simulink model "Application_Problem_Solution"  (R2018b)
settings: Solver=VariableStepAuto  StartTime=0.0  StopTime=6300  FixedStep=0.1  RelTol=1e-3  EnableMultiTasking=on
StopFcn:
  | if sum(Diagnostic_Decision_PV_1)>0
  | f = msgbox('Failure in PV 1');
  | end
  | 
  | if sum(Diagnostic_Decision_PV_2)>0
  | f = msgbox('Failure in PV 2');
  | end
  | 
  | if sum(Diagnostic_Decision_PV_3)>0
  | f = msgbox('Failure in PV 3');
  | end
  | 
  | if sum(Diagnostic_Decision_PV_4)>0
  | f = msgbox('Failure in PV 4');
  | end
  | 
  | if sum(Diagnostic_Decision_PV_5)>0
  | f = msgbox('Failure in PV 5');
  | end
  | 
  | if sum(Diagnostic_Decision_PV_6)>0
  | f = msgbox('Failure in PV 6');
  | end
  | 
  | if sum(Diagnostic_Decision_PV_7)>0
  | f = msgbox('Failure in PV 7');
  | end
  | 
  | if sum(Diagnostic_Decision_PV_8)>0
  | f = msgbox('Failure in PV 8');
  | end
  | 
  | if sum(Diagnostic_Decision_PV_9)>0
  | f = msgbox('Failure in PV 9');
  | end
  | 
  | if sum(Diagnostic_Decision_PV_10)>0
  | f = msgbox('Failure in PV 10');
  | end
values from neighbouring files (symbols this model uses):
  C1_LUT = [1913.6 4625.7 23306 10736 18036 12251 9022.9 12447 18872 40764 18721 33630 ... (21 elements, 7x3)]    [model_data_application.mat]
  Capacity_LUT = [28.0081 27.625 27.6392]    [model_data_application.mat]
  cell_Cp_heat = 810.5328    [model_data_application.mat]
  cell_mass = 1    [model_data_application.mat]
  Em_LUT = [3.4966 3.5519 3.6183 3.7066 3.9131 4.0748 4.1923 3.5057 3.566 3.6337 3.7127 3.9259 ... (21 elements, 7x3)]    [model_data_application.mat]
  Qe_init = 3.6845    [model_data_application.mat]
  R0_LUT = [0.0117 0.011 0.0114 0.0107 0.0107 0.0113 0.0116 0.0085 0.0085 0.0087 0.0082 0.0083 ... (21 elements, 7x3)]    [model_data_application.mat]
  R1_LUT = [0.0109 0.0069 0.0047 0.0034 0.0033 0.0033 0.0028 0.0029 0.0024 0.0026 0.0016 0.0023 ... (21 elements, 7x3)]    [model_data_application.mat]
  SOC_LUT = [0 0.1 0.25 0.5 0.75 0.9 1]    [model_data_application.mat]
  T_init = 293.15    [model_data_application.mat]
  Temperature_LUT = [278.15 293.15 313.15]    [model_data_application.mat]
undefined symbols (not defined in the file or in its folder): DiscIntNeverNeededParam
libraries: elec_lib x450, fl_lib x121, LiBatteryElements_lib x40, nesl_utility x32, simulink x10
(part 2 of 3)

== system Application_Problem_Solution/Battery7 ==
  C1 : LiBatteryElements_lib/C_table  C_Table=C1_LUT F  SOC_Table=SOC_LUT  Temp_Table=Temperature_LUT K  v0=0 V
  Convective Heat Transfer : fl_lib/Thermal/Thermal Elements/Convective Heat Transfer  area=cell_area m^2  heat_tr_coeff=h_conv W/(m^2 * K)  T_specify=off  T_priority=High  T=0 K  T_nominal_specify=off  T_nominal_unit=K  T_nominal_value=1  Q_specify=off  Q_priority=High  Q=0 J/s  Q_nominal_specify=off  Q_nominal_unit=W  Q_nominal_value=1
  Em_table : LiBatteryElements_lib/Em_table  C_Table=Capacity_LUT hr*A  Em_Table=Em_LUT V  SOC_Table=SOC_LUT  Temp_Table=Temperature_LUT K  Qinit=Qe_init hr*A
  Ideal Temperature Source : fl_lib/Thermal/Thermal Sources/Controlled Temperature Source
      settings: SourceProductName=Simscape
  Power Sum : fl_lib/Physical Signals/Functions/PS Add
  R0 : LiBatteryElements_lib/R_table  R_Table=R0_LUT Ohm  SOC_Table=SOC_LUT  Temp_Table=Temperature_LUT K
  R1 : LiBatteryElements_lib/R_table  R_Table=R1_LUT Ohm  SOC_Table=SOC_LUT  Temp_Table=Temperature_LUT K
  Simulink-PS Converter2 : nesl_utility/Simulink-PS Converter  PhysicalDomain=network_engine_domain  SubClassName=ps_input  LeftPortType=input  RightPortType=output  PseudoPeriodic=off  Frequencies=[]  NoiseDistribution=none  NoiseParameters=[]  Unit=degC  AffineConversion=on  FilteringAndDerivatives=zero  SimscapeFilterOrder=1  InputFilterTimeConstant=.001  UdotUserProvided=1
  Thermal Model : Subsystem
  Thermal Reference : fl_lib/Thermal/Thermal Elements/Thermal Reference
  temp : Constant  Value=25
  + : PMIOPort  Tag=PMCPort  Side=Left
  - : PMIOPort  Tag=PMCPort  Port=2  Side=Right
  wires:
  temp/1 -> Simulink-PS Converter2/1
  connections:
  Thermal Reference/LConn1 -- Ideal Temperature Source/RConn2
  Ideal Temperature Source/LConn1 -- Convective Heat Transfer/LConn1
  Simulink-PS Converter2/RConn1 -- Ideal Temperature Source/RConn1
  R0/RConn2 -- Power Sum/LConn1
  R0/LConn1 -- C1/RConn1 -- R1/RConn1
  Power Sum/RConn1 -- Thermal Model/LConn1
  C1/LConn2 -- R0/LConn2 -- Em_table/RConn2 -- Thermal Model/RConn1 -- R1/LConn2
  R1/RConn2 -- Power Sum/LConn2
  R1/LConn1 -- C1/LConn1 -- Em_table/LConn1
  +/RConn1 -- R0/RConn1
  Em_table/RConn1 -- -/RConn1
  Convective Heat Transfer/RConn1 -- Thermal Model/LConn2
  C1/LConn3 -- Em_table/LConn3 -- R0/LConn3 -- R1/LConn3

== system Application_Problem_Solution/Battery8 ==
  C1 : LiBatteryElements_lib/C_table  C_Table=C1_LUT F  SOC_Table=SOC_LUT  Temp_Table=Temperature_LUT K  v0=0 V
  Convective Heat Transfer : fl_lib/Thermal/Thermal Elements/Convective Heat Transfer  area=cell_area m^2  heat_tr_coeff=h_conv W/(m^2 * K)  T_specify=off  T_priority=High  T=0 K  T_nominal_specify=off  T_nominal_unit=K  T_nominal_value=1  Q_specify=off  Q_priority=High  Q=0 J/s  Q_nominal_specify=off  Q_nominal_unit=W  Q_nominal_value=1
  Em_table : LiBatteryElements_lib/Em_table  C_Table=Capacity_LUT hr*A  Em_Table=Em_LUT V  SOC_Table=SOC_LUT  Temp_Table=Temperature_LUT K  Qinit=Qe_init hr*A
  Ideal Temperature Source : fl_lib/Thermal/Thermal Sources/Controlled Temperature Source
      settings: SourceProductName=Simscape
  Power Sum : fl_lib/Physical Signals/Functions/PS Add
  R0 : LiBatteryElements_lib/R_table  R_Table=R0_LUT Ohm  SOC_Table=SOC_LUT  Temp_Table=Temperature_LUT K
  R1 : LiBatteryElements_lib/R_table  R_Table=R1_LUT Ohm  SOC_Table=SOC_LUT  Temp_Table=Temperature_LUT K
  Simulink-PS Converter2 : nesl_utility/Simulink-PS Converter  PhysicalDomain=network_engine_domain  SubClassName=ps_input  LeftPortType=input  RightPortType=output  PseudoPeriodic=off  Frequencies=[]  NoiseDistribution=none  NoiseParameters=[]  Unit=degC  AffineConversion=on  FilteringAndDerivatives=zero  SimscapeFilterOrder=1  InputFilterTimeConstant=.001  UdotUserProvided=1
  Thermal Model : Subsystem
  Thermal Reference : fl_lib/Thermal/Thermal Elements/Thermal Reference
  temp : Constant  Value=25
  + : PMIOPort  Tag=PMCPort  Side=Left
  - : PMIOPort  Tag=PMCPort  Port=2  Side=Right
  wires:
  temp/1 -> Simulink-PS Converter2/1
  connections:
  R1/LConn3 -- R0/LConn3 -- Em_table/LConn3 -- C1/LConn3
  Convective Heat Transfer/RConn1 -- Thermal Model/LConn2
  Em_table/RConn1 -- -/RConn1
  +/RConn1 -- R0/RConn1
  Em_table/LConn1 -- C1/LConn1 -- R1/LConn1
  R1/RConn2 -- Power Sum/LConn2
  R1/LConn2 -- Thermal Model/RConn1 -- Em_table/RConn2 -- R0/LConn2 -- C1/LConn2
  Power Sum/RConn1 -- Thermal Model/LConn1
  R1/RConn1 -- C1/RConn1 -- R0/LConn1
  R0/RConn2 -- Power Sum/LConn1
  Simulink-PS Converter2/RConn1 -- Ideal Temperature Source/RConn1
  Ideal Temperature Source/LConn1 -- Convective Heat Transfer/LConn1
  Thermal Reference/LConn1 -- Ideal Temperature Source/RConn2

== system Application_Problem_Solution/Battery9 ==
  C1 : LiBatteryElements_lib/C_table  C_Table=C1_LUT F  SOC_Table=SOC_LUT  Temp_Table=Temperature_LUT K  v0=0 V
  Convective Heat Transfer : fl_lib/Thermal/Thermal Elements/Convective Heat Transfer  area=cell_area m^2  heat_tr_coeff=h_conv W/(m^2 * K)  T_specify=off  T_priority=High  T=0 K  T_nominal_specify=off  T_nominal_unit=K  T_nominal_value=1  Q_specify=off  Q_priority=High  Q=0 J/s  Q_nominal_specify=off  Q_nominal_unit=W  Q_nominal_value=1
  Em_table : LiBatteryElements_lib/Em_table  C_Table=Capacity_LUT hr*A  Em_Table=Em_LUT V  SOC_Table=SOC_LUT  Temp_Table=Temperature_LUT K  Qinit=Qe_init hr*A
  Ideal Temperature Source : fl_lib/Thermal/Thermal Sources/Controlled Temperature Source
      settings: SourceProductName=Simscape
  Power Sum : fl_lib/Physical Signals/Functions/PS Add
  R0 : LiBatteryElements_lib/R_table  R_Table=R0_LUT Ohm  SOC_Table=SOC_LUT  Temp_Table=Temperature_LUT K
  R1 : LiBatteryElements_lib/R_table  R_Table=R1_LUT Ohm  SOC_Table=SOC_LUT  Temp_Table=Temperature_LUT K
  Simulink-PS Converter2 : nesl_utility/Simulink-PS Converter  PhysicalDomain=network_engine_domain  SubClassName=ps_input  LeftPortType=input  RightPortType=output  PseudoPeriodic=off  Frequencies=[]  NoiseDistribution=none  NoiseParameters=[]  Unit=degC  AffineConversion=on  FilteringAndDerivatives=zero  SimscapeFilterOrder=1  InputFilterTimeConstant=.001  UdotUserProvided=1
  Thermal Model : Subsystem
  Thermal Reference : fl_lib/Thermal/Thermal Elements/Thermal Reference
  temp : Constant  Value=25
  + : PMIOPort  Tag=PMCPort  Side=Left
  - : PMIOPort  Tag=PMCPort  Port=2  Side=Right
  wires:
  temp/1 -> Simulink-PS Converter2/1
  connections:
  Thermal Reference/LConn1 -- Ideal Temperature Source/RConn2
  Ideal Temperature Source/LConn1 -- Convective Heat Transfer/LConn1
  Simulink-PS Converter2/RConn1 -- Ideal Temperature Source/RConn1
  R0/RConn2 -- Power Sum/LConn1
  R0/LConn1 -- C1/RConn1 -- R1/RConn1
  Power Sum/RConn1 -- Thermal Model/LConn1
  C1/LConn2 -- R0/LConn2 -- Em_table/RConn2 -- Thermal Model/RConn1 -- R1/LConn2
  R1/RConn2 -- Power Sum/LConn2
  R1/LConn1 -- C1/LConn1 -- Em_table/LConn1
  +/RConn1 -- R0/RConn1
  Em_table/RConn1 -- -/RConn1
  Convective Heat Transfer/RConn1 -- Thermal Model/LConn2
  C1/LConn3 -- Em_table/LConn3 -- R0/LConn3 -- R1/LConn3

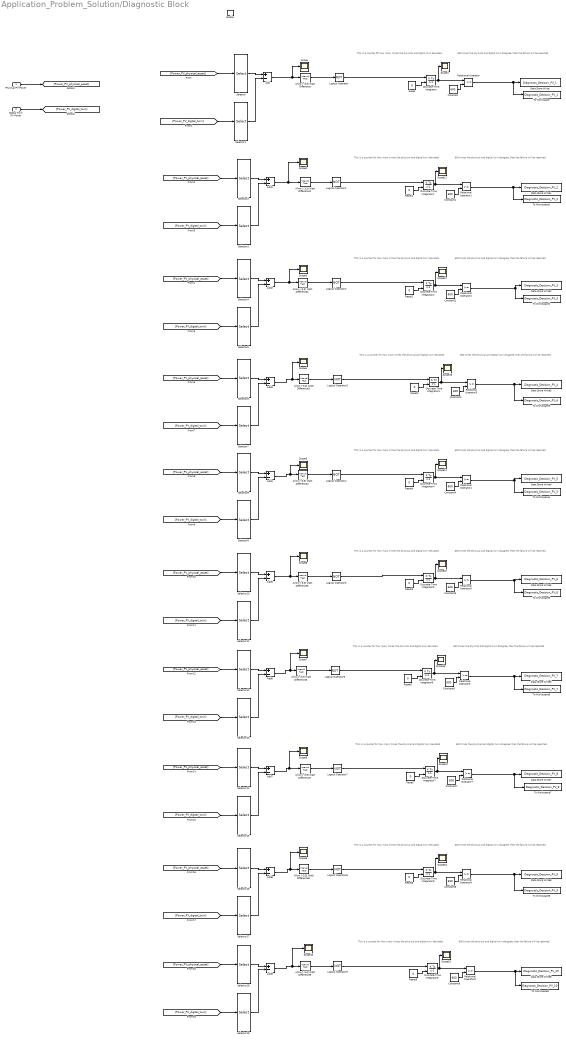
== system Application_Problem_Solution/Diagnostic Block ==
  note: 600 times the physical and digital twin disagree, then the failure will be reported.
  note: This is a counter for how many times the physical and digital twin deviated.
  note: 600 times the physical and digital twin disagree, then the failure will be reported.
  note: This is a counter for how many times the physical and digital twin deviated.
  note: 600 times the physical and digital twin disagree, then the failure will be reported.
  note: This is a counter for how many times the physical and digital twin deviated.
  note: 600 times the physical and digital twin disagree, then the failure will be reported.
  note: This is a counter for how many times the physical and digital twin deviated.
  note: 600 times the physical and digital twin disagree, then the failure will be reported.
  note: This is a counter for how many times the physical and digital twin deviated.
  note: 600 times the physical and digital twin disagree, then the failure will be reported.
  note: This is a counter for how many times the physical and digital twin deviated.
  note: 600 times the physical and digital twin disagree, then the failure will be reported.
  note: This is a counter for how many times the physical and digital twin deviated.
  note: 600 times the physical and digital twin disagree, then the failure will be reported.
  note: This is a counter for how many times the physical and digital twin deviated.
  note: 600 times the physical and digital twin disagree, then the failure will be reported.
  note: This is a counter for how many times the physical and digital twin deviated.
  note: 600 times the physical and digital twin disagree, then the failure will be reported.
  note: This is a counter for how many times the physical and digital twin deviated.
  Physical PV-Power : Inport
  Digital Twin PV-Power : Inport  Port=2
  Enable : EnablePort
  Add{,1..9} (10 alike) : Sum  Inputs=+-
  Allow [-3,3] Watt Difference{,1..9} (10 alike) : simulink/Logic and Bit Operations/Interval Test  IntervalClosedRight=on  uplimit=3  IntervalClosedLeft=on  lowlimit=-3  OutDataTypeStr=boolean
  Constant{,1..9} (10 alike) : Constant  Value=600
  Data Store Write : DataStoreWrite  DataStoreName=Diagnostic_Decision_PV_1  SampleTime=10
  Data Store Write1 : DataStoreWrite  DataStoreName=Diagnostic_Decision_PV_2  SampleTime=100
  Data Store Write2 : DataStoreWrite  DataStoreName=Diagnostic_Decision_PV_3  SampleTime=10
  Data Store Write3 : DataStoreWrite  DataStoreName=Diagnostic_Decision_PV_4  SampleTime=10
  Data Store Write4 : DataStoreWrite  DataStoreName=Diagnostic_Decision_PV_5  SampleTime=10
  Data Store Write5 : DataStoreWrite  DataStoreName=Diagnostic_Decision_PV_6
  Data Store Write6 : DataStoreWrite  DataStoreName=Diagnostic_Decision_PV_7  SampleTime=10
  Data Store Write7 : DataStoreWrite  DataStoreName=Diagnostic_Decision_PV_8  SampleTime=10
  Data Store Write8 : DataStoreWrite  DataStoreName=Diagnostic_Decision_PV_9  SampleTime=10
  Data Store Write9 : DataStoreWrite  DataStoreName=Diagnostic_Decision_PV_10  SampleTime=10
  Discrete-Time Integrator : DiscreteIntegrator  ExternalReset=rising  SampleTime=10  ICPrevOutput=DiscIntNeverNeededParam  ICPrevScaledInput=DiscIntNeverNeededParam
  Discrete-Time Integrator{1..9} (9 alike) : DiscreteIntegrator  ExternalReset=level  SampleTime=10  ICPrevOutput=DiscIntNeverNeededParam  ICPrevScaledInput=DiscIntNeverNeededParam
  Logical Operator{,1..9} (10 alike) : Logic  Operator=NOT  AllPortsSameDT=off  OutDataTypeStr=boolean
  Relational Operator{,1..9} (10 alike) : RelationalOperator  OutDataTypeStr=boolean  RndMeth=Simplest
  Reset{,1..9} (10 alike) : Constant  Value=0
  Scope{,1..19} (20 alike) : Scope
  Selector : Selector  InputPortWidth=10  IndexOptions=Index vector (dialog)  Indices=1  OutputSizes=1
  Selector1 : Selector  InputPortWidth=10  IndexOptions=Index vector (dialog)  Indices=1  OutputSizes=1
  Selector{10..13} (4 alike) : Selector  InputPortWidth=10  IndexOptions=Index vector (dialog)  Indices=6  OutputSizes=1
  Selector14 : Selector  InputPortWidth=10  IndexOptions=Index vector (dialog)  Indices=8  OutputSizes=1
  Selector15 : Selector  InputPortWidth=10  IndexOptions=Index vector (dialog)  Indices=8  OutputSizes=1
  Selector16 : Selector  InputPortWidth=10  IndexOptions=Index vector (dialog)  Indices=9  OutputSizes=1
  Selector17 : Selector  InputPortWidth=10  IndexOptions=Index vector (dialog)  Indices=9  OutputSizes=1
  Selector18 : Selector  InputPortWidth=10  IndexOptions=Index vector (dialog)  Indices=10  OutputSizes=1
  Selector19 : Selector  InputPortWidth=10  IndexOptions=Index vector (dialog)  Indices=10  OutputSizes=1
  Selector2 : Selector  InputPortWidth=10  IndexOptions=Index vector (dialog)  Indices=2  OutputSizes=1
  Selector3 : Selector  InputPortWidth=10  IndexOptions=Index vector (dialog)  Indices=2  OutputSizes=1
  Selector4 : Selector  InputPortWidth=10  IndexOptions=Index vector (dialog)  Indices=3  OutputSizes=1
  Selector5 : Selector  InputPortWidth=10  IndexOptions=Index vector (dialog)  Indices=3  OutputSizes=1
  Selector6 : Selector  InputPortWidth=10  IndexOptions=Index vector (dialog)  Indices=4  OutputSizes=1
  Selector7 : Selector  InputPortWidth=10  IndexOptions=Index vector (dialog)  Indices=4  OutputSizes=1
  Selector8 : Selector  InputPortWidth=10  IndexOptions=Index vector (dialog)  Indices=5  OutputSizes=1
  Selector9 : Selector  InputPortWidth=10  IndexOptions=Index vector (dialog)  Indices=5  OutputSizes=1
  To Workspace : ToWorkspace  VariableName=Diagnostic_Decision_PV_1  SampleTime=10
  To Workspace1 : ToWorkspace  VariableName=Diagnostic_Decision_PV_2  SampleTime=10
  To Workspace2 : ToWorkspace  VariableName=Diagnostic_Decision_PV_3  SampleTime=10
  To Workspace3 : ToWorkspace  VariableName=Diagnostic_Decision_PV_4  SampleTime=10
  To Workspace4 : ToWorkspace  VariableName=Diagnostic_Decision_PV_5  SampleTime=10
  To Workspace5 : ToWorkspace  VariableName=Diagnostic_Decision_PV_6  SampleTime=10
  To Workspace6 : ToWorkspace  VariableName=Diagnostic_Decision_PV_7  SampleTime=10
  To Workspace7 : ToWorkspace  VariableName=Diagnostic_Decision_PV_8  SampleTime=10
  To Workspace8 : ToWorkspace  VariableName=Diagnostic_Decision_PV_9  SampleTime=10
  To Workspace9 : ToWorkspace  VariableName=Diagnostic_Decision_PV_10  SampleTime=10
  wires:
  Physical PV-Power/1 -> [Power_PV_physical_asset]
  Digital Twin PV-Power/1 -> [Power_PV_digital_twin]
  [Power_PV_physical_asset] -> Selector/1
  [Power_PV_digital_twin] -> Selector1/1
  Selector/1 -> Add/1
  Selector1/1 -> Add/2
  Discrete-Time Integrator/1 -> Scope1/1, Relational Operator/1
  Constant/1 -> Relational Operator/2
  Relational Operator/1 -> To Workspace/1, Data Store Write/1
  Selector3/1 -> Add1/2
  Selector2/1 -> Add1/1
  [Power_PV_digital_twin] -> Selector3/1
  [Power_PV_physical_asset] -> Selector2/1
  [Power_PV_physical_asset] -> Selector4/1
  [Power_PV_digital_twin] -> Selector5/1
  Selector4/1 -> Add2/1
  Selector5/1 -> Add2/2
  Selector7/1 -> Add3/2
  Selector6/1 -> Add3/1
  [Power_PV_digital_twin] -> Selector7/1
  [Power_PV_physical_asset] -> Selector6/1
  [Power_PV_physical_asset] -> Selector8/1
  [Power_PV_digital_twin] -> Selector9/1
  Selector8/1 -> Add4/1
  Selector9/1 -> Add4/2
  Selector11/1 -> Add5/2
  Selector10/1 -> Add5/1
  [Power_PV_digital_twin] -> Selector11/1
  [Power_PV_physical_asset] -> Selector10/1
  [Power_PV_physical_asset] -> Selector12/1
  [Power_PV_digital_twin] -> Selector13/1
  Selector12/1 -> Add6/1
  Selector13/1 -> Add6/2
  Selector15/1 -> Add7/2
  Selector14/1 -> Add7/1
  [Power_PV_digital_twin] -> Selector15/1
  [Power_PV_physical_asset] -> Selector14/1
  [Power_PV_physical_asset] -> Selector16/1
  [Power_PV_digital_twin] -> Selector17/1
  Selector16/1 -> Add8/1
  Selector17/1 -> Add8/2
  Selector19/1 -> Add9/2
  Selector18/1 -> Add9/1
  [Power_PV_digital_twin] -> Selector19/1
  [Power_PV_physical_asset] -> Selector18/1
  Add/1 -> Scope/1, Allow [-3,3] Watt Difference/1
  Allow [-3,3] Watt Difference/1 -> Logical Operator/1
  Logical Operator/1 -> Discrete-Time Integrator/1
  Allow [-3,3] Watt Difference1/1 -> Logical Operator1/1
  Add1/1 -> Allow [-3,3] Watt Difference1/1, Scope2/1
  Add2/1 -> Allow [-3,3] Watt Difference2/1, Scope3/1
  Allow [-3,3] Watt Difference2/1 -> Logical Operator2/1
  Add3/1 -> Allow [-3,3] Watt Difference3/1, Scope4/1
  Allow [-3,3] Watt Difference3/1 -> Logical Operator3/1
  Add4/1 -> Scope5/1, Allow [-3,3] Watt Difference4/1
  Allow [-3,3] Watt Difference4/1 -> Logical Operator4/1
  Add5/1 -> Allow [-3,3] Watt Difference5/1, Scope6/1
  Allow [-3,3] Watt Difference5/1 -> Logical Operator5/1
  Add6/1 -> Scope7/1, Allow [-3,3] Watt Difference6/1
  Allow [-3,3] Watt Difference6/1 -> Logical Operator6/1
  Add7/1 -> Allow [-3,3] Watt Difference7/1, Scope8/1
  Allow [-3,3] Watt Difference7/1 -> Logical Operator7/1
  Add8/1 -> Allow [-3,3] Watt Difference8/1, Scope9/1
  Allow [-3,3] Watt Difference8/1 -> Logical Operator8/1
  Add9/1 -> Allow [-3,3] Watt Difference9/1, Scope10/1
  Allow [-3,3] Watt Difference9/1 -> Logical Operator9/1
  Reset/1 -> Discrete-Time Integrator/2
  Discrete-Time Integrator1/1 -> Scope11/1, Relational Operator1/1
  Logical Operator1/1 -> Discrete-Time Integrator1/1
  Constant1/1 -> Relational Operator1/2
  Reset1/1 -> Discrete-Time Integrator1/2
  Relational Operator1/1 -> To Workspace1/1, Data Store Write1/1
  Discrete-Time Integrator2/1 -> Scope12/1, Relational Operator2/1
  Logical Operator2/1 -> Discrete-Time Integrator2/1
  Constant2/1 -> Relational Operator2/2
  Reset2/1 -> Discrete-Time Integrator2/2
  Relational Operator2/1 -> Data Store Write2/1, To Workspace2/1
  Discrete-Time Integrator3/1 -> Scope13/1, Relational Operator3/1
  Logical Operator3/1 -> Discrete-Time Integrator3/1
  Constant3/1 -> Relational Operator3/2
  Reset3/1 -> Discrete-Time Integrator3/2
  Relational Operator3/1 -> Data Store Write3/1, To Workspace3/1
  Discrete-Time Integrator4/1 -> Scope14/1, Relational Operator4/1
  Logical Operator4/1 -> Discrete-Time Integrator4/1
  Constant4/1 -> Relational Operator4/2
  Reset4/1 -> Discrete-Time Integrator4/2
  Relational Operator4/1 -> Data Store Write4/1, To Workspace4/1
  Discrete-Time Integrator5/1 -> Scope15/1, Relational Operator5/1
  Logical Operator5/1 -> Discrete-Time Integrator5/1
  Constant5/1 -> Relational Operator5/2
  Reset5/1 -> Discrete-Time Integrator5/2
  Relational Operator5/1 -> Data Store Write5/1, To Workspace5/1
  Discrete-Time Integrator6/1 -> Scope16/1, Relational Operator6/1
  Logical Operator6/1 -> Discrete-Time Integrator6/1
  Constant6/1 -> Relational Operator6/2
  Reset6/1 -> Discrete-Time Integrator6/2
  Relational Operator6/1 -> To Workspace6/1, Data Store Write6/1
  Discrete-Time Integrator7/1 -> Scope17/1, Relational Operator7/1
  Logical Operator7/1 -> Discrete-Time Integrator7/1
  Constant7/1 -> Relational Operator7/2
  Reset7/1 -> Discrete-Time Integrator7/2
  Relational Operator7/1 -> To Workspace7/1, Data Store Write7/1
  Discrete-Time Integrator8/1 -> Scope18/1, Relational Operator8/1
  Logical Operator8/1 -> Discrete-Time Integrator8/1
  Constant8/1 -> Relational Operator8/2
  Reset8/1 -> Discrete-Time Integrator8/2
  Relational Operator8/1 -> To Workspace8/1, Data Store Write8/1
  Discrete-Time Integrator9/1 -> Scope19/1, Relational Operator9/1
  Logical Operator9/1 -> Discrete-Time Integrator9/1
  Constant9/1 -> Relational Operator9/2
  Reset9/1 -> Discrete-Time Integrator9/2
  Relational Operator9/1 -> Data Store Write9/1, To Workspace9/1

== system Application_Problem_Solution/PV 1 Physical ==
  note: 'This is a dummy model for the physical system. It is used for display reasons. Data has been pre-generated.'
  In1 : Inport
  Power_PV1_physical_asset : FromWorkspace  VariableName=Power_PV1_physical_asset  SampleTime=0
  Terminator : Terminator
  Out1 : Outport
  wires:
  In1/1 -> Terminator/1
  Power_PV1_physical_asset/1 -> Out1/1

== system Application_Problem_Solution/PV 10 Physical ==
  note: 'This is a dummy model for the physical system. It is used for display reasons. Data has been pre-generated.'
  In1 : Inport
  Power_PV1_physical_asset : FromWorkspace  VariableName=Power_PV10_physical_asset  SampleTime=0
  Terminator : Terminator
  Out1 : Outport
  wires:
  Power_PV1_physical_asset/1 -> Out1/1
  In1/1 -> Terminator/1

== system Application_Problem_Solution/PV 2 Physical  ==
  note: 'This is a dummy model for the physical system. It is used for display reasons. Data has been pre-generated.'
  In1 : Inport
  Power_PV2_physical_asset : FromWorkspace  VariableName=Power_PV2_physical_asset  SampleTime=0
  Terminator : Terminator
  Out1 : Outport
  wires:
  Power_PV2_physical_asset/1 -> Out1/1
  In1/1 -> Terminator/1

== system Application_Problem_Solution/PV 3 Physical ==
  note: 'This is a dummy model for the physical system. It is used for display reasons. Data has been pre-generated.'
  In1 : Inport
  Power_PV3_physical_asset : FromWorkspace  VariableName=Power_PV3_physical_asset  SampleTime=0
  Terminator : Terminator
  Out1 : Outport
  wires:
  In1/1 -> Terminator/1
  Power_PV3_physical_asset/1 -> Out1/1

== system Application_Problem_Solution/PV 4 Physical ==
  note: 'This is a dummy model for the physical system. It is used for display reasons. Data has been pre-generated.'
  In1 : Inport
  Power_PV4_physical_asset : FromWorkspace  VariableName=Power_PV4_physical_asset  SampleTime=0
  Terminator : Terminator
  Out1 : Outport
  wires:
  Power_PV4_physical_asset/1 -> Out1/1
  In1/1 -> Terminator/1

== system Application_Problem_Solution/PV 5 Physical ==
  note: 'This is a dummy model for the physical system. It is used for display reasons. Data has been pre-generated.'
  In1 : Inport
  Power_PV5_physical_asset : FromWorkspace  VariableName=Power_PV5_physical_asset  SampleTime=0
  Terminator : Terminator
  Out1 : Outport
  wires:
  In1/1 -> Terminator/1
  Power_PV5_physical_asset/1 -> Out1/1

== system Application_Problem_Solution/PV 6 Physical ==
  note: 'This is a dummy model for the physical system. It is used for display reasons. Data has been pre-generated.'
  In1 : Inport
  Power_PV6_physical_asset : FromWorkspace  VariableName=Power_PV6_physical_asset  SampleTime=0
  Terminator : Terminator
  Out1 : Outport
  wires:
  Power_PV6_physical_asset/1 -> Out1/1
  In1/1 -> Terminator/1

== system Application_Problem_Solution/PV 7 Physical ==
  note: 'This is a dummy model for the physical system. It is used for display reasons. Data has been pre-generated.'
  In1 : Inport
  Power_PV7_physical_asset : FromWorkspace  VariableName=Power_PV7_physical_asset  SampleTime=0
  Terminator : Terminator
  Out1 : Outport
  wires:
  In1/1 -> Terminator/1
  Power_PV7_physical_asset/1 -> Out1/1

== system Application_Problem_Solution/PV 8 Physical ==
  note: 'This is a dummy model for the physical system. It is used for display reasons. Data has been pre-generated.'
  In1 : Inport
  Power_PV1_physical_asset : FromWorkspace  VariableName=Power_PV8_physical_asset  SampleTime=0
  Terminator : Terminator
  Out1 : Outport
  wires:
  Power_PV1_physical_asset/1 -> Out1/1
  In1/1 -> Terminator/1

== system Application_Problem_Solution/PV 9 Physical ==
  note: 'This is a dummy model for the physical system. It is used for display reasons. Data has been pre-generated.'
  In1 : Inport
  Power_PV1_physical_asset : FromWorkspace  VariableName=Power_PV9_physical_asset  SampleTime=0
  Terminator : Terminator
  Out1 : Outport
  wires:
  In1/1 -> Terminator/1
  Power_PV1_physical_asset/1 -> Out1/1

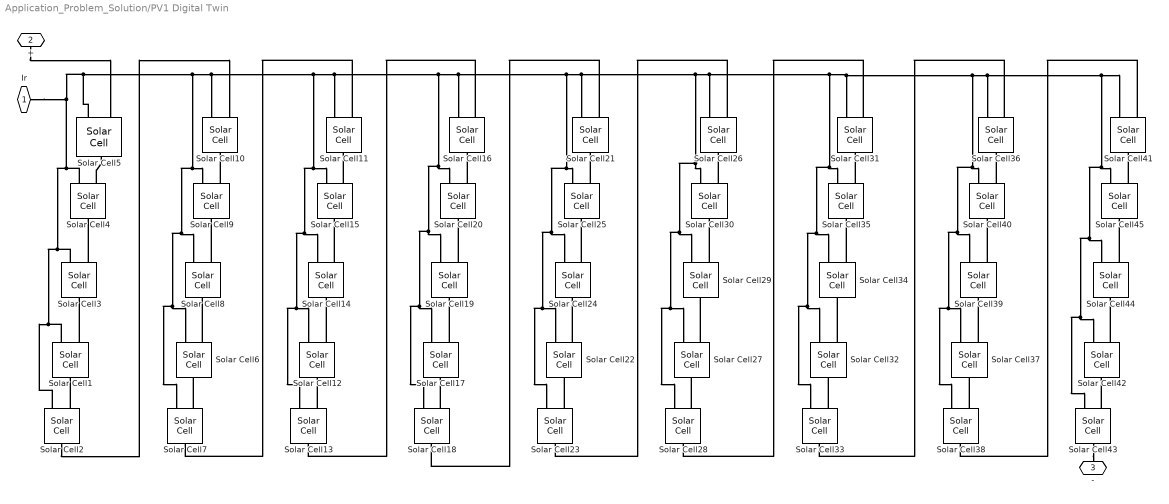
== system Application_Problem_Solution/PV1 Digital Twin ==
  Solar Cell{1..45} (45 alike) : elec_lib/Sources/Solar Cell  prm=1  Isc=Isc A  Voc=Voc/45 V  Is=1e-6 A  Is2=0 A  Iph=7.34 A  Ir0=Ir0 W/m^2  ec=n  N2=2  Rs=Rs/45 Ohm  Rp=Inf Ohm  N_series=1  TIPH1=0 1/K  EG=1.11 eV  TXIS1=3  TXIS2=3  TRS1=0  TRP1=0  Tmeas=T degC  TFIXED=T degC  thermal_mass=100 J/K  initial_temperature=25 degC
      settings: SourceProductName=Simscape Electronics  SourceProductBaseCode=SN
  Ir : PMIOPort  Side=Left
  + : PMIOPort  Port=2  Side=Right
  - : PMIOPort  Port=3  Side=Right
  connections:
  Solar Cell5/LConn1 -- Solar Cell7/LConn1 -- Solar Cell6/LConn1 -- Solar Cell8/LConn1 -- Solar Cell9/LConn1 -- Solar Cell13/LConn1 -- Solar Cell12/LConn1 -- Solar Cell14/LConn1 -- Solar Cell15/LConn1 -- Solar Cell18/LConn1 -- Solar Cell17/LConn1 -- Solar Cell19/LConn1 -- Solar Cell20/LConn1 -- Solar Cell22/LConn1 -- Solar Cell23/LConn1 -- Solar Cell24/LConn1 -- Solar Cell25/LConn1 -- Solar Cell28/LConn1 -- Solar Cell27/LConn1 -- Solar Cell29/LConn1 -- Solar Cell30/LConn1 -- Solar Cell33/LConn1 -- Solar Cell32/LConn1 -- Solar Cell34/LConn1 -- Solar Cell35/LConn1 -- Solar Cell37/LConn1 -- Solar Cell38/LConn1 -- Solar Cell39/LConn1 -- Solar Cell40/LConn1 -- Solar Cell43/LConn1 -- Solar Cell42/LConn1 -- Solar Cell44/LConn1 -- Solar Cell45/LConn1 -- Solar Cell41/LConn1 -- Solar Cell36/LConn1 -- Solar Cell31/LConn1 -- Solar Cell26/LConn1 -- Solar Cell21/LConn1 -- Solar Cell16/LConn1 -- Solar Cell11/LConn1 -- Solar Cell10/LConn1 -- Solar Cell4/LConn1 -- Solar Cell3/LConn1 -- Solar Cell1/LConn1 -- Solar Cell2/LConn1 -- Ir/RConn1
  Solar Cell3/LConn2 -- Solar Cell4/RConn1
  Solar Cell2/LConn2 -- Solar Cell1/RConn1
  Solar Cell1/LConn2 -- Solar Cell3/RConn1
  Solar Cell4/LConn2 -- Solar Cell5/RConn1
  +/RConn1 -- Solar Cell5/LConn2
  Solar Cell9/LConn2 -- Solar Cell10/RConn1
  Solar Cell7/LConn2 -- Solar Cell6/RConn1
  Solar Cell6/LConn2 -- Solar Cell8/RConn1
  Solar Cell2/RConn1 -- Solar Cell10/LConn2
  Solar Cell8/LConn2 -- Solar Cell9/RConn1
  Solar Cell11/LConn2 -- Solar Cell7/RConn1
  Solar Cell12/LConn2 -- Solar Cell14/RConn1
  Solar Cell13/LConn2 -- Solar Cell12/RConn1
  Solar Cell15/LConn2 -- Solar Cell11/RConn1
  Solar Cell14/LConn2 -- Solar Cell15/RConn1
  Solar Cell19/LConn2 -- Solar Cell20/RConn1
  Solar Cell20/LConn2 -- Solar Cell16/RConn1
  Solar Cell16/LConn2 -- Solar Cell13/RConn1
  Solar Cell17/LConn2 -- Solar Cell19/RConn1
  Solar Cell18/LConn2 -- Solar Cell17/RConn1
  Solar Cell23/LConn2 -- Solar Cell22/RConn1
  Solar Cell22/LConn2 -- Solar Cell24/RConn1
  Solar Cell25/LConn2 -- Solar Cell21/RConn1
  Solar Cell21/LConn2 -- Solar Cell18/RConn1
  Solar Cell24/LConn2 -- Solar Cell25/RConn1
  Solar Cell29/LConn2 -- Solar Cell30/RConn1
  Solar Cell26/LConn2 -- Solar Cell23/RConn1
  Solar Cell30/LConn2 -- Solar Cell26/RConn1
  Solar Cell27/LConn2 -- Solar Cell29/RConn1
  Solar Cell28/LConn2 -- Solar Cell27/RConn1
  Solar Cell34/LConn2 -- Solar Cell35/RConn1
  Solar Cell31/LConn2 -- Solar Cell28/RConn1
  Solar Cell35/LConn2 -- Solar Cell31/RConn1
  Solar Cell32/LConn2 -- Solar Cell34/RConn1
  Solar Cell33/LConn2 -- Solar Cell32/RConn1
  Solar Cell39/LConn2 -- Solar Cell40/RConn1
  Solar Cell36/LConn2 -- Solar Cell33/RConn1
  Solar Cell40/LConn2 -- Solar Cell36/RConn1
  Solar Cell37/LConn2 -- Solar Cell39/RConn1
  Solar Cell38/LConn2 -- Solar Cell37/RConn1
  Solar Cell44/LConn2 -- Solar Cell45/RConn1
  Solar Cell41/LConn2 -- Solar Cell38/RConn1
  Solar Cell45/LConn2 -- Solar Cell41/RConn1
  Solar Cell42/LConn2 -- Solar Cell44/RConn1
  Solar Cell43/LConn2 -- Solar Cell42/RConn1
  Solar Cell43/RConn1 -- -/RConn1

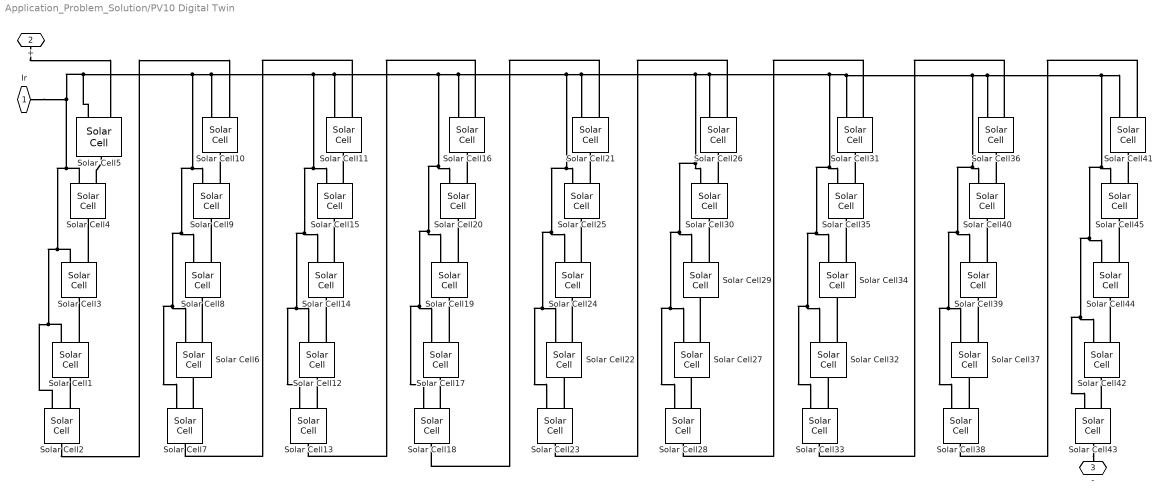
== system Application_Problem_Solution/PV10 Digital Twin ==
  Solar Cell{1..45} (45 alike) : elec_lib/Sources/Solar Cell  prm=1  Isc=Isc A  Voc=Voc/45 V  Is=1e-6 A  Is2=0 A  Iph=7.34 A  Ir0=Ir0 W/m^2  ec=n  N2=2  Rs=Rs/45 Ohm  Rp=Inf Ohm  N_series=1  TIPH1=0 1/K  EG=1.11 eV  TXIS1=3  TXIS2=3  TRS1=0  TRP1=0  Tmeas=T degC  TFIXED=T degC  thermal_mass=100 J/K  initial_temperature=25 degC
      settings: SourceProductName=Simscape Electronics  SourceProductBaseCode=SN
  Ir : PMIOPort  Side=Left
  + : PMIOPort  Port=2  Side=Right
  - : PMIOPort  Port=3  Side=Right
  connections:
  Solar Cell43/RConn1 -- -/RConn1
  Solar Cell43/LConn2 -- Solar Cell42/RConn1
  Solar Cell42/LConn2 -- Solar Cell44/RConn1
  Solar Cell45/LConn2 -- Solar Cell41/RConn1
  Solar Cell41/LConn2 -- Solar Cell38/RConn1
  Solar Cell44/LConn2 -- Solar Cell45/RConn1
  Solar Cell38/LConn2 -- Solar Cell37/RConn1
  Solar Cell37/LConn2 -- Solar Cell39/RConn1
  Solar Cell40/LConn2 -- Solar Cell36/RConn1
  Solar Cell36/LConn2 -- Solar Cell33/RConn1
  Solar Cell39/LConn2 -- Solar Cell40/RConn1
  Solar Cell33/LConn2 -- Solar Cell32/RConn1
  Solar Cell32/LConn2 -- Solar Cell34/RConn1
  Solar Cell35/LConn2 -- Solar Cell31/RConn1
  Solar Cell31/LConn2 -- Solar Cell28/RConn1
  Solar Cell34/LConn2 -- Solar Cell35/RConn1
  Solar Cell28/LConn2 -- Solar Cell27/RConn1
  Solar Cell27/LConn2 -- Solar Cell29/RConn1
  Solar Cell30/LConn2 -- Solar Cell26/RConn1
  Solar Cell26/LConn2 -- Solar Cell23/RConn1
  Solar Cell29/LConn2 -- Solar Cell30/RConn1
  Solar Cell24/LConn2 -- Solar Cell25/RConn1
  Solar Cell21/LConn2 -- Solar Cell18/RConn1
  Solar Cell25/LConn2 -- Solar Cell21/RConn1
  Solar Cell22/LConn2 -- Solar Cell24/RConn1
  Solar Cell23/LConn2 -- Solar Cell22/RConn1
  Solar Cell18/LConn2 -- Solar Cell17/RConn1
  Solar Cell17/LConn2 -- Solar Cell19/RConn1
  Solar Cell16/LConn2 -- Solar Cell13/RConn1
  Solar Cell20/LConn2 -- Solar Cell16/RConn1
  Solar Cell19/LConn2 -- Solar Cell20/RConn1
  Solar Cell14/LConn2 -- Solar Cell15/RConn1
  Solar Cell15/LConn2 -- Solar Cell11/RConn1
  Solar Cell13/LConn2 -- Solar Cell12/RConn1
  Solar Cell12/LConn2 -- Solar Cell14/RConn1
  Solar Cell11/LConn2 -- Solar Cell7/RConn1
  Solar Cell8/LConn2 -- Solar Cell9/RConn1
  Solar Cell2/RConn1 -- Solar Cell10/LConn2
  Solar Cell6/LConn2 -- Solar Cell8/RConn1
  Solar Cell7/LConn2 -- Solar Cell6/RConn1
  Solar Cell9/LConn2 -- Solar Cell10/RConn1
  +/RConn1 -- Solar Cell5/LConn2
  Solar Cell4/LConn2 -- Solar Cell5/RConn1
  Solar Cell1/LConn2 -- Solar Cell3/RConn1
  Solar Cell2/LConn2 -- Solar Cell1/RConn1
  Solar Cell3/LConn2 -- Solar Cell4/RConn1
  Ir/RConn1 -- Solar Cell2/LConn1 -- Solar Cell1/LConn1 -- Solar Cell3/LConn1 -- Solar Cell4/LConn1 -- Solar Cell10/LConn1 -- Solar Cell11/LConn1 -- Solar Cell16/LConn1 -- Solar Cell21/LConn1 -- Solar Cell26/LConn1 -- Solar Cell31/LConn1 -- Solar Cell36/LConn1 -- Solar Cell41/LConn1 -- Solar Cell45/LConn1 -- Solar Cell44/LConn1 -- Solar Cell42/LConn1 -- Solar Cell43/LConn1 -- Solar Cell40/LConn1 -- Solar Cell39/LConn1 -- Solar Cell38/LConn1 -- Solar Cell37/LConn1 -- Solar Cell35/LConn1 -- Solar Cell34/LConn1 -- Solar Cell32/LConn1 -- Solar Cell33/LConn1 -- Solar Cell30/LConn1 -- Solar Cell29/LConn1 -- Solar Cell27/LConn1 -- Solar Cell28/LConn1 -- Solar Cell25/LConn1 -- Solar Cell24/LConn1 -- Solar Cell23/LConn1 -- Solar Cell22/LConn1 -- Solar Cell20/LConn1 -- Solar Cell19/LConn1 -- Solar Cell17/LConn1 -- Solar Cell18/LConn1 -- Solar Cell15/LConn1 -- Solar Cell14/LConn1 -- Solar Cell12/LConn1 -- Solar Cell13/LConn1 -- Solar Cell9/LConn1 -- Solar Cell8/LConn1 -- Solar Cell6/LConn1 -- Solar Cell7/LConn1 -- Solar Cell5/LConn1

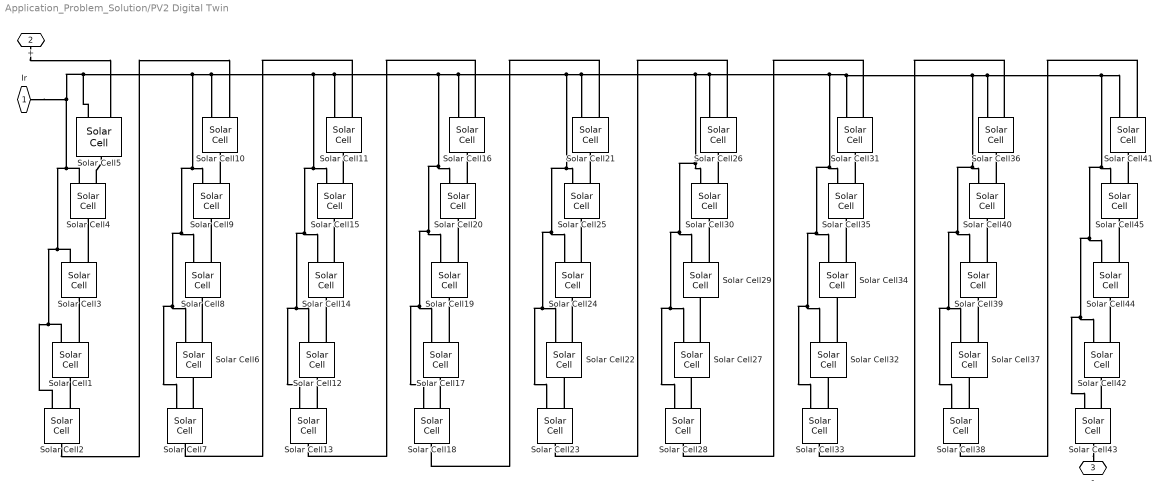
== system Application_Problem_Solution/PV2 Digital Twin ==
  Solar Cell{1..45} (45 alike) : elec_lib/Sources/Solar Cell  prm=1  Isc=Isc A  Voc=Voc/45 V  Is=1e-6 A  Is2=0 A  Iph=7.34 A  Ir0=Ir0 W/m^2  ec=n  N2=2  Rs=Rs/45 Ohm  Rp=Inf Ohm  N_series=1  TIPH1=0 1/K  EG=1.11 eV  TXIS1=3  TXIS2=3  TRS1=0  TRP1=0  Tmeas=T degC  TFIXED=T degC  thermal_mass=100 J/K  initial_temperature=25 degC
      settings: SourceProductName=Simscape Electronics  SourceProductBaseCode=SN
  Ir : PMIOPort  Side=Left
  + : PMIOPort  Port=2  Side=Right
  - : PMIOPort  Port=3  Side=Right
  connections:
  Solar Cell43/RConn1 -- -/RConn1
  Solar Cell43/LConn2 -- Solar Cell42/RConn1
  Solar Cell42/LConn2 -- Solar Cell44/RConn1
  Solar Cell45/LConn2 -- Solar Cell41/RConn1
  Solar Cell41/LConn2 -- Solar Cell38/RConn1
  Solar Cell44/LConn2 -- Solar Cell45/RConn1
  Solar Cell38/LConn2 -- Solar Cell37/RConn1
  Solar Cell37/LConn2 -- Solar Cell39/RConn1
  Solar Cell40/LConn2 -- Solar Cell36/RConn1
  Solar Cell36/LConn2 -- Solar Cell33/RConn1
  Solar Cell39/LConn2 -- Solar Cell40/RConn1
  Solar Cell33/LConn2 -- Solar Cell32/RConn1
  Solar Cell32/LConn2 -- Solar Cell34/RConn1
  Solar Cell35/LConn2 -- Solar Cell31/RConn1
  Solar Cell31/LConn2 -- Solar Cell28/RConn1
  Solar Cell34/LConn2 -- Solar Cell35/RConn1
  Solar Cell28/LConn2 -- Solar Cell27/RConn1
  Solar Cell27/LConn2 -- Solar Cell29/RConn1
  Solar Cell30/LConn2 -- Solar Cell26/RConn1
  Solar Cell26/LConn2 -- Solar Cell23/RConn1
  Solar Cell29/LConn2 -- Solar Cell30/RConn1
  Solar Cell24/LConn2 -- Solar Cell25/RConn1
  Solar Cell21/LConn2 -- Solar Cell18/RConn1
  Solar Cell25/LConn2 -- Solar Cell21/RConn1
  Solar Cell22/LConn2 -- Solar Cell24/RConn1
  Solar Cell23/LConn2 -- Solar Cell22/RConn1
  Solar Cell18/LConn2 -- Solar Cell17/RConn1
  Solar Cell17/LConn2 -- Solar Cell19/RConn1
  Solar Cell16/LConn2 -- Solar Cell13/RConn1
  Solar Cell20/LConn2 -- Solar Cell16/RConn1
  Solar Cell19/LConn2 -- Solar Cell20/RConn1
  Solar Cell14/LConn2 -- Solar Cell15/RConn1
  Solar Cell15/LConn2 -- Solar Cell11/RConn1
  Solar Cell13/LConn2 -- Solar Cell12/RConn1
  Solar Cell12/LConn2 -- Solar Cell14/RConn1
  Solar Cell11/LConn2 -- Solar Cell7/RConn1
  Solar Cell8/LConn2 -- Solar Cell9/RConn1
  Solar Cell2/RConn1 -- Solar Cell10/LConn2
  Solar Cell6/LConn2 -- Solar Cell8/RConn1
  Solar Cell7/LConn2 -- Solar Cell6/RConn1
  Solar Cell9/LConn2 -- Solar Cell10/RConn1
  +/RConn1 -- Solar Cell5/LConn2
  Solar Cell4/LConn2 -- Solar Cell5/RConn1
  Solar Cell1/LConn2 -- Solar Cell3/RConn1
  Solar Cell2/LConn2 -- Solar Cell1/RConn1
  Solar Cell3/LConn2 -- Solar Cell4/RConn1
  Ir/RConn1 -- Solar Cell2/LConn1 -- Solar Cell1/LConn1 -- Solar Cell3/LConn1 -- Solar Cell4/LConn1 -- Solar Cell10/LConn1 -- Solar Cell11/LConn1 -- Solar Cell16/LConn1 -- Solar Cell21/LConn1 -- Solar Cell26/LConn1 -- Solar Cell31/LConn1 -- Solar Cell36/LConn1 -- Solar Cell41/LConn1 -- Solar Cell45/LConn1 -- Solar Cell44/LConn1 -- Solar Cell42/LConn1 -- Solar Cell43/LConn1 -- Solar Cell40/LConn1 -- Solar Cell39/LConn1 -- Solar Cell38/LConn1 -- Solar Cell37/LConn1 -- Solar Cell35/LConn1 -- Solar Cell34/LConn1 -- Solar Cell32/LConn1 -- Solar Cell33/LConn1 -- Solar Cell30/LConn1 -- Solar Cell29/LConn1 -- Solar Cell27/LConn1 -- Solar Cell28/LConn1 -- Solar Cell25/LConn1 -- Solar Cell24/LConn1 -- Solar Cell23/LConn1 -- Solar Cell22/LConn1 -- Solar Cell20/LConn1 -- Solar Cell19/LConn1 -- Solar Cell17/LConn1 -- Solar Cell18/LConn1 -- Solar Cell15/LConn1 -- Solar Cell14/LConn1 -- Solar Cell12/LConn1 -- Solar Cell13/LConn1 -- Solar Cell9/LConn1 -- Solar Cell8/LConn1 -- Solar Cell6/LConn1 -- Solar Cell7/LConn1 -- Solar Cell5/LConn1

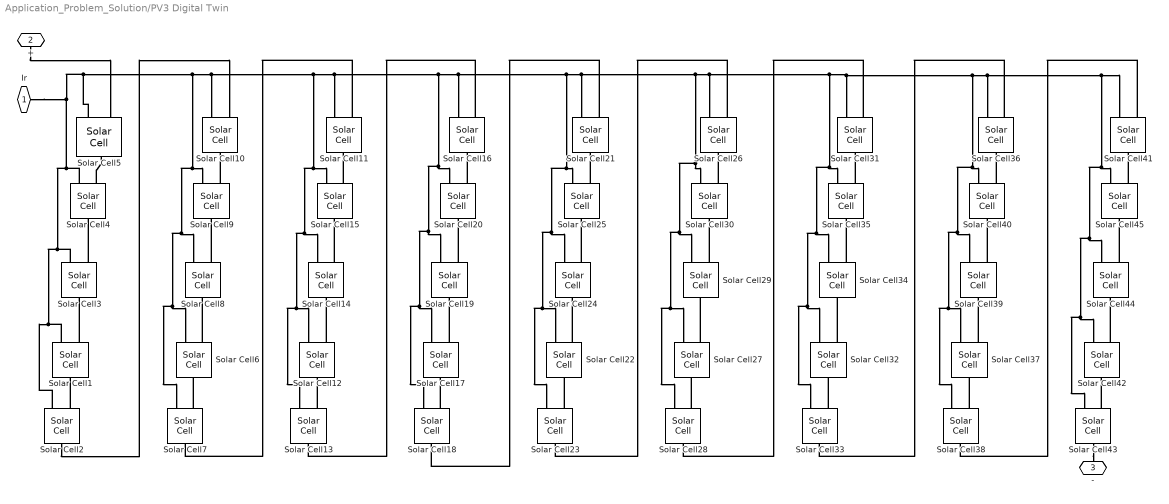
== system Application_Problem_Solution/PV3 Digital Twin  ==
  Solar Cell{1..45} (45 alike) : elec_lib/Sources/Solar Cell  prm=1  Isc=Isc A  Voc=Voc/45 V  Is=1e-6 A  Is2=0 A  Iph=7.34 A  Ir0=Ir0 W/m^2  ec=n  N2=2  Rs=Rs/45 Ohm  Rp=Inf Ohm  N_series=1  TIPH1=0 1/K  EG=1.11 eV  TXIS1=3  TXIS2=3  TRS1=0  TRP1=0  Tmeas=T degC  TFIXED=T degC  thermal_mass=100 J/K  initial_temperature=25 degC
      settings: SourceProductName=Simscape Electronics  SourceProductBaseCode=SN
  Ir : PMIOPort  Side=Left
  + : PMIOPort  Port=2  Side=Right
  - : PMIOPort  Port=3  Side=Right
  connections:
  Solar Cell5/LConn1 -- Solar Cell7/LConn1 -- Solar Cell6/LConn1 -- Solar Cell8/LConn1 -- Solar Cell9/LConn1 -- Solar Cell13/LConn1 -- Solar Cell12/LConn1 -- Solar Cell14/LConn1 -- Solar Cell15/LConn1 -- Solar Cell18/LConn1 -- Solar Cell17/LConn1 -- Solar Cell19/LConn1 -- Solar Cell20/LConn1 -- Solar Cell22/LConn1 -- Solar Cell23/LConn1 -- Solar Cell24/LConn1 -- Solar Cell25/LConn1 -- Solar Cell28/LConn1 -- Solar Cell27/LConn1 -- Solar Cell29/LConn1 -- Solar Cell30/LConn1 -- Solar Cell33/LConn1 -- Solar Cell32/LConn1 -- Solar Cell34/LConn1 -- Solar Cell35/LConn1 -- Solar Cell37/LConn1 -- Solar Cell38/LConn1 -- Solar Cell39/LConn1 -- Solar Cell40/LConn1 -- Solar Cell43/LConn1 -- Solar Cell42/LConn1 -- Solar Cell44/LConn1 -- Solar Cell45/LConn1 -- Solar Cell41/LConn1 -- Solar Cell36/LConn1 -- Solar Cell31/LConn1 -- Solar Cell26/LConn1 -- Solar Cell21/LConn1 -- Solar Cell16/LConn1 -- Solar Cell11/LConn1 -- Solar Cell10/LConn1 -- Solar Cell4/LConn1 -- Solar Cell3/LConn1 -- Solar Cell1/LConn1 -- Solar Cell2/LConn1 -- Ir/RConn1
  Solar Cell3/LConn2 -- Solar Cell4/RConn1
  Solar Cell2/LConn2 -- Solar Cell1/RConn1
  Solar Cell1/LConn2 -- Solar Cell3/RConn1
  Solar Cell4/LConn2 -- Solar Cell5/RConn1
  +/RConn1 -- Solar Cell5/LConn2
  Solar Cell9/LConn2 -- Solar Cell10/RConn1
  Solar Cell7/LConn2 -- Solar Cell6/RConn1
  Solar Cell6/LConn2 -- Solar Cell8/RConn1
  Solar Cell2/RConn1 -- Solar Cell10/LConn2
  Solar Cell8/LConn2 -- Solar Cell9/RConn1
  Solar Cell11/LConn2 -- Solar Cell7/RConn1
  Solar Cell12/LConn2 -- Solar Cell14/RConn1
  Solar Cell13/LConn2 -- Solar Cell12/RConn1
  Solar Cell15/LConn2 -- Solar Cell11/RConn1
  Solar Cell14/LConn2 -- Solar Cell15/RConn1
  Solar Cell19/LConn2 -- Solar Cell20/RConn1
  Solar Cell20/LConn2 -- Solar Cell16/RConn1
  Solar Cell16/LConn2 -- Solar Cell13/RConn1
  Solar Cell17/LConn2 -- Solar Cell19/RConn1
  Solar Cell18/LConn2 -- Solar Cell17/RConn1
  Solar Cell23/LConn2 -- Solar Cell22/RConn1
  Solar Cell22/LConn2 -- Solar Cell24/RConn1
  Solar Cell25/LConn2 -- Solar Cell21/RConn1
  Solar Cell21/LConn2 -- Solar Cell18/RConn1
  Solar Cell24/LConn2 -- Solar Cell25/RConn1
  Solar Cell29/LConn2 -- Solar Cell30/RConn1
  Solar Cell26/LConn2 -- Solar Cell23/RConn1
  Solar Cell30/LConn2 -- Solar Cell26/RConn1
  Solar Cell27/LConn2 -- Solar Cell29/RConn1
  Solar Cell28/LConn2 -- Solar Cell27/RConn1
  Solar Cell34/LConn2 -- Solar Cell35/RConn1
  Solar Cell31/LConn2 -- Solar Cell28/RConn1
  Solar Cell35/LConn2 -- Solar Cell31/RConn1
  Solar Cell32/LConn2 -- Solar Cell34/RConn1
  Solar Cell33/LConn2 -- Solar Cell32/RConn1
  Solar Cell39/LConn2 -- Solar Cell40/RConn1
  Solar Cell36/LConn2 -- Solar Cell33/RConn1
  Solar Cell40/LConn2 -- Solar Cell36/RConn1
  Solar Cell37/LConn2 -- Solar Cell39/RConn1
  Solar Cell38/LConn2 -- Solar Cell37/RConn1
  Solar Cell44/LConn2 -- Solar Cell45/RConn1
  Solar Cell41/LConn2 -- Solar Cell38/RConn1
  Solar Cell45/LConn2 -- Solar Cell41/RConn1
  Solar Cell42/LConn2 -- Solar Cell44/RConn1
  Solar Cell43/LConn2 -- Solar Cell42/RConn1
  Solar Cell43/RConn1 -- -/RConn1

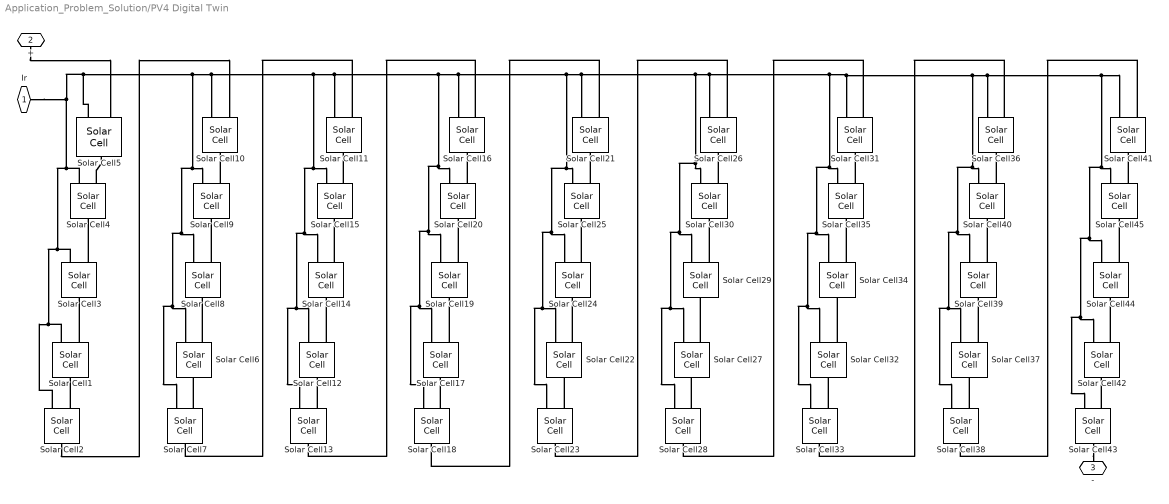
== system Application_Problem_Solution/PV4 Digital Twin ==
  Solar Cell{1..45} (45 alike) : elec_lib/Sources/Solar Cell  prm=1  Isc=Isc A  Voc=Voc/45 V  Is=1e-6 A  Is2=0 A  Iph=7.34 A  Ir0=Ir0 W/m^2  ec=n  N2=2  Rs=Rs/45 Ohm  Rp=Inf Ohm  N_series=1  TIPH1=0 1/K  EG=1.11 eV  TXIS1=3  TXIS2=3  TRS1=0  TRP1=0  Tmeas=T degC  TFIXED=T degC  thermal_mass=100 J/K  initial_temperature=25 degC
      settings: SourceProductName=Simscape Electronics  SourceProductBaseCode=SN
  Ir : PMIOPort  Side=Left
  + : PMIOPort  Port=2  Side=Right
  - : PMIOPort  Port=3  Side=Right
  connections:
  Solar Cell43/RConn1 -- -/RConn1
  Solar Cell43/LConn2 -- Solar Cell42/RConn1
  Solar Cell42/LConn2 -- Solar Cell44/RConn1
  Solar Cell45/LConn2 -- Solar Cell41/RConn1
  Solar Cell41/LConn2 -- Solar Cell38/RConn1
  Solar Cell44/LConn2 -- Solar Cell45/RConn1
  Solar Cell38/LConn2 -- Solar Cell37/RConn1
  Solar Cell37/LConn2 -- Solar Cell39/RConn1
  Solar Cell40/LConn2 -- Solar Cell36/RConn1
  Solar Cell36/LConn2 -- Solar Cell33/RConn1
  Solar Cell39/LConn2 -- Solar Cell40/RConn1
  Solar Cell33/LConn2 -- Solar Cell32/RConn1
  Solar Cell32/LConn2 -- Solar Cell34/RConn1
  Solar Cell35/LConn2 -- Solar Cell31/RConn1
  Solar Cell31/LConn2 -- Solar Cell28/RConn1
  Solar Cell34/LConn2 -- Solar Cell35/RConn1
  Solar Cell28/LConn2 -- Solar Cell27/RConn1
  Solar Cell27/LConn2 -- Solar Cell29/RConn1
  Solar Cell30/LConn2 -- Solar Cell26/RConn1
  Solar Cell26/LConn2 -- Solar Cell23/RConn1
  Solar Cell29/LConn2 -- Solar Cell30/RConn1
  Solar Cell24/LConn2 -- Solar Cell25/RConn1
  Solar Cell21/LConn2 -- Solar Cell18/RConn1
  Solar Cell25/LConn2 -- Solar Cell21/RConn1
  Solar Cell22/LConn2 -- Solar Cell24/RConn1
  Solar Cell23/LConn2 -- Solar Cell22/RConn1
  Solar Cell18/LConn2 -- Solar Cell17/RConn1
  Solar Cell17/LConn2 -- Solar Cell19/RConn1
  Solar Cell16/LConn2 -- Solar Cell13/RConn1
  Solar Cell20/LConn2 -- Solar Cell16/RConn1
  Solar Cell19/LConn2 -- Solar Cell20/RConn1
  Solar Cell14/LConn2 -- Solar Cell15/RConn1
  Solar Cell15/LConn2 -- Solar Cell11/RConn1
  Solar Cell13/LConn2 -- Solar Cell12/RConn1
  Solar Cell12/LConn2 -- Solar Cell14/RConn1
  Solar Cell11/LConn2 -- Solar Cell7/RConn1
  Solar Cell8/LConn2 -- Solar Cell9/RConn1
  Solar Cell2/RConn1 -- Solar Cell10/LConn2
  Solar Cell6/LConn2 -- Solar Cell8/RConn1
  Solar Cell7/LConn2 -- Solar Cell6/RConn1
  Solar Cell9/LConn2 -- Solar Cell10/RConn1
  +/RConn1 -- Solar Cell5/LConn2
  Solar Cell4/LConn2 -- Solar Cell5/RConn1
  Solar Cell1/LConn2 -- Solar Cell3/RConn1
  Solar Cell2/LConn2 -- Solar Cell1/RConn1
  Solar Cell3/LConn2 -- Solar Cell4/RConn1
  Ir/RConn1 -- Solar Cell2/LConn1 -- Solar Cell1/LConn1 -- Solar Cell3/LConn1 -- Solar Cell4/LConn1 -- Solar Cell10/LConn1 -- Solar Cell11/LConn1 -- Solar Cell16/LConn1 -- Solar Cell21/LConn1 -- Solar Cell26/LConn1 -- Solar Cell31/LConn1 -- Solar Cell36/LConn1 -- Solar Cell41/LConn1 -- Solar Cell45/LConn1 -- Solar Cell44/LConn1 -- Solar Cell42/LConn1 -- Solar Cell43/LConn1 -- Solar Cell40/LConn1 -- Solar Cell39/LConn1 -- Solar Cell38/LConn1 -- Solar Cell37/LConn1 -- Solar Cell35/LConn1 -- Solar Cell34/LConn1 -- Solar Cell32/LConn1 -- Solar Cell33/LConn1 -- Solar Cell30/LConn1 -- Solar Cell29/LConn1 -- Solar Cell27/LConn1 -- Solar Cell28/LConn1 -- Solar Cell25/LConn1 -- Solar Cell24/LConn1 -- Solar Cell23/LConn1 -- Solar Cell22/LConn1 -- Solar Cell20/LConn1 -- Solar Cell19/LConn1 -- Solar Cell17/LConn1 -- Solar Cell18/LConn1 -- Solar Cell15/LConn1 -- Solar Cell14/LConn1 -- Solar Cell12/LConn1 -- Solar Cell13/LConn1 -- Solar Cell9/LConn1 -- Solar Cell8/LConn1 -- Solar Cell6/LConn1 -- Solar Cell7/LConn1 -- Solar Cell5/LConn1

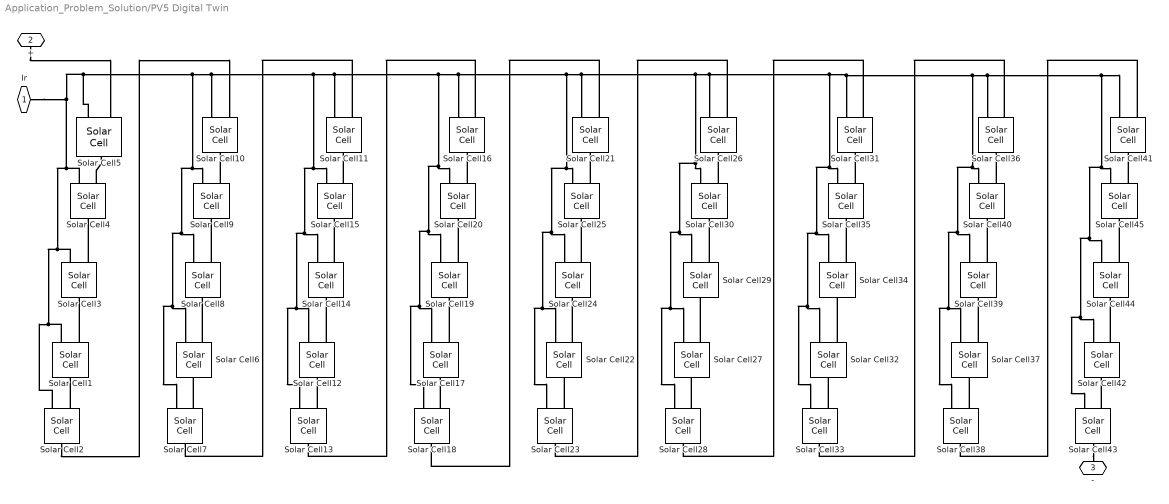
== system Application_Problem_Solution/PV5 Digital Twin ==
  Solar Cell{1..45} (45 alike) : elec_lib/Sources/Solar Cell  prm=1  Isc=Isc A  Voc=Voc/45 V  Is=1e-6 A  Is2=0 A  Iph=7.34 A  Ir0=Ir0 W/m^2  ec=n  N2=2  Rs=Rs/45 Ohm  Rp=Inf Ohm  N_series=1  TIPH1=0 1/K  EG=1.11 eV  TXIS1=3  TXIS2=3  TRS1=0  TRP1=0  Tmeas=T degC  TFIXED=T degC  thermal_mass=100 J/K  initial_temperature=25 degC
      settings: SourceProductName=Simscape Electronics  SourceProductBaseCode=SN
  Ir : PMIOPort  Side=Left
  + : PMIOPort  Port=2  Side=Right
  - : PMIOPort  Port=3  Side=Right
  connections:
  Solar Cell5/LConn1 -- Solar Cell7/LConn1 -- Solar Cell6/LConn1 -- Solar Cell8/LConn1 -- Solar Cell9/LConn1 -- Solar Cell13/LConn1 -- Solar Cell12/LConn1 -- Solar Cell14/LConn1 -- Solar Cell15/LConn1 -- Solar Cell18/LConn1 -- Solar Cell17/LConn1 -- Solar Cell19/LConn1 -- Solar Cell20/LConn1 -- Solar Cell22/LConn1 -- Solar Cell23/LConn1 -- Solar Cell24/LConn1 -- Solar Cell25/LConn1 -- Solar Cell28/LConn1 -- Solar Cell27/LConn1 -- Solar Cell29/LConn1 -- Solar Cell30/LConn1 -- Solar Cell33/LConn1 -- Solar Cell32/LConn1 -- Solar Cell34/LConn1 -- Solar Cell35/LConn1 -- Solar Cell37/LConn1 -- Solar Cell38/LConn1 -- Solar Cell39/LConn1 -- Solar Cell40/LConn1 -- Solar Cell43/LConn1 -- Solar Cell42/LConn1 -- Solar Cell44/LConn1 -- Solar Cell45/LConn1 -- Solar Cell41/LConn1 -- Solar Cell36/LConn1 -- Solar Cell31/LConn1 -- Solar Cell26/LConn1 -- Solar Cell21/LConn1 -- Solar Cell16/LConn1 -- Solar Cell11/LConn1 -- Solar Cell10/LConn1 -- Solar Cell4/LConn1 -- Solar Cell3/LConn1 -- Solar Cell1/LConn1 -- Solar Cell2/LConn1 -- Ir/RConn1
  Solar Cell3/LConn2 -- Solar Cell4/RConn1
  Solar Cell2/LConn2 -- Solar Cell1/RConn1
  Solar Cell1/LConn2 -- Solar Cell3/RConn1
  Solar Cell4/LConn2 -- Solar Cell5/RConn1
  +/RConn1 -- Solar Cell5/LConn2
  Solar Cell9/LConn2 -- Solar Cell10/RConn1
  Solar Cell7/LConn2 -- Solar Cell6/RConn1
  Solar Cell6/LConn2 -- Solar Cell8/RConn1
  Solar Cell2/RConn1 -- Solar Cell10/LConn2
  Solar Cell8/LConn2 -- Solar Cell9/RConn1
  Solar Cell11/LConn2 -- Solar Cell7/RConn1
  Solar Cell12/LConn2 -- Solar Cell14/RConn1
  Solar Cell13/LConn2 -- Solar Cell12/RConn1
  Solar Cell15/LConn2 -- Solar Cell11/RConn1
  Solar Cell14/LConn2 -- Solar Cell15/RConn1
  Solar Cell19/LConn2 -- Solar Cell20/RConn1
  Solar Cell20/LConn2 -- Solar Cell16/RConn1
  Solar Cell16/LConn2 -- Solar Cell13/RConn1
  Solar Cell17/LConn2 -- Solar Cell19/RConn1
  Solar Cell18/LConn2 -- Solar Cell17/RConn1
  Solar Cell23/LConn2 -- Solar Cell22/RConn1
  Solar Cell22/LConn2 -- Solar Cell24/RConn1
  Solar Cell25/LConn2 -- Solar Cell21/RConn1
  Solar Cell21/LConn2 -- Solar Cell18/RConn1
  Solar Cell24/LConn2 -- Solar Cell25/RConn1
  Solar Cell29/LConn2 -- Solar Cell30/RConn1
  Solar Cell26/LConn2 -- Solar Cell23/RConn1
  Solar Cell30/LConn2 -- Solar Cell26/RConn1
  Solar Cell27/LConn2 -- Solar Cell29/RConn1
  Solar Cell28/LConn2 -- Solar Cell27/RConn1
  Solar Cell34/LConn2 -- Solar Cell35/RConn1
  Solar Cell31/LConn2 -- Solar Cell28/RConn1
  Solar Cell35/LConn2 -- Solar Cell31/RConn1
  Solar Cell32/LConn2 -- Solar Cell34/RConn1
  Solar Cell33/LConn2 -- Solar Cell32/RConn1
  Solar Cell39/LConn2 -- Solar Cell40/RConn1
  Solar Cell36/LConn2 -- Solar Cell33/RConn1
  Solar Cell40/LConn2 -- Solar Cell36/RConn1
  Solar Cell37/LConn2 -- Solar Cell39/RConn1
  Solar Cell38/LConn2 -- Solar Cell37/RConn1
  Solar Cell44/LConn2 -- Solar Cell45/RConn1
  Solar Cell41/LConn2 -- Solar Cell38/RConn1
  Solar Cell45/LConn2 -- Solar Cell41/RConn1
  Solar Cell42/LConn2 -- Solar Cell44/RConn1
  Solar Cell43/LConn2 -- Solar Cell42/RConn1
  Solar Cell43/RConn1 -- -/RConn1
